simulink model "TestRoomVolume"  (R2025b)
settings: Solver=daessc  StartTime=0.0  StopTime=7200  FixedStep=3600  MaxStep=3  RelTol=1e-3  AbsTol=1e-3
PreLoadFcn:
  | WallModelParams
libraries: fl_lib x3, nesl_utility x2, buildingEnergy_lib x1
CloseFcn:
  | clear flow out roomHeight wall win
settings Model: Creator=vikrants  LastModifiedBy=skota
settings SolverCC: AutoScaleAbsTol=off  AlgebraicLoopSolver=TrustRegion  MaxZcPerStep=1.0
settings DebuggingCC: UnconnectedInputMsg=warning  UnconnectedOutputMsg=warning  UnconnectedLineMsg=warning  SymbolicDimsDataTypeCodeGenerationDiagnostic=none
settings ModelReferenceCC: EnableRefExpFcnMdlSchedulingChecks=on
settings SFSimCC: CustomCodeUndefinedFunction=UseInterfaceOnly
settings RTWCC: GPUComputeCapability=3.5  DLArmComputeVersion=19.05
settings SimscapeCC: SimscapeLogType=all  SimscapeLogSimulationStatistics=on  SimscapeLogDataHistory=10000.0

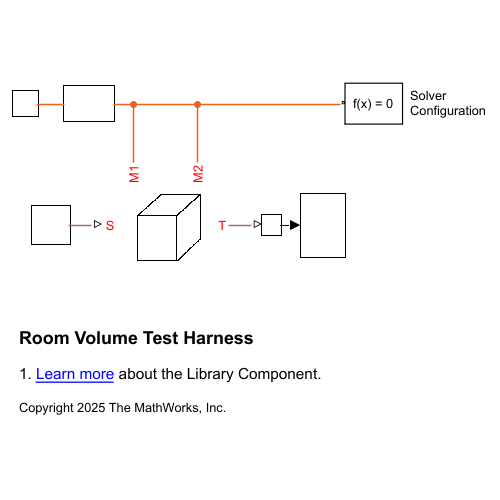
[thumbnail: Simulink's stored preview of the top-level diagram]
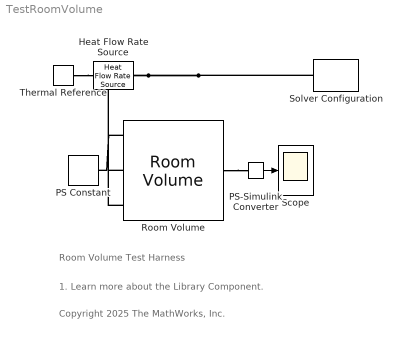
== system TestRoomVolume ==
  note: Room Volume Test Harness
  note: 1. Learn more about the Library Component.
  note: Copyright 2025 The MathWorks, Inc.
  Heat Flow Rate Source : fl_lib/Thermal/Thermal Sources/Heat Flow Rate Source  heat_flow=100 W
  PS Constant : fl_lib/Physical Signals/Sources/PS Constant  constant=100 J/s
  PS-Simulink Converter : nesl_utility/PS-Simulink Converter  PhysicalDomain=network_engine_domain  SubClassName=ps_output  LeftPortType=input  RightPortType=output  PseudoPeriodic=off  Frequencies=[]  VectorFormat=inherit  Unit=inherit  AffineConversion=off
  Room Volume : buildingEnergy_lib/Room Volume  N1=1  N2=1  iniT=300 K  length=5 m  width=3 m  height=2.5 m
  Scope : Scope
      settings: ActiveDisplayYMinimum=294.54266386219956  ActiveDisplayYMaximum=349.11602524020395
  Solver Configuration : nesl_utility/Solver Configuration  PhysicalDomain=network_engine_domain  SubClassName=solver  LeftPortType=input  RightPortType=generic  Tones=[]  Harmonics=[]  SimulateNoise=off  Profile=off  UseLocalSampling=off  EnableSwitchedLinearOptims=on  FrequencyDomain=off  UseCCode=off  RelTol=0.001  AbsTol=1e-06  MinStep=1e-09  ToWorkspace=off  RevertToSquareIcSolve=off  NumHomotopyIterations=100  PhasorMode=off  PhasorModeNumHarmonics=1  ConsistencySolver=NEWTON_XTOL_AFTER_FTOL  CanonicalOrdering=UNORDERED  OptimizeIntermediates=UNOPTIMIZED  IndexReductionMethod=DerivativeReplacement  DoDC=off  ResidualTolerance=1e-09  ConsistencyTolSource=GLOBAL  ConsistencyAbsTol=0.001  ConsistencyRelTol=0.001  ConsistencyTolFactor=0.001  UseLocalSolver=off  LocalSolverChoice=NE_BACKWARD_EULER_ADVANCER  ResolveIndetEquations=on  FunctionEvalNumThread=1  LocalSolverSampleTime=0.001  DoFixedCost=off  MaxNonlinIter=3  MaxModeIter=2  ComputeImpulses=off  ImpulseIterations=2  LinearAlgebra=auto  LinearAlgebraNumThread=0  EquationFormulation=NE_TIME_EF  DelaysMemoryBudget=1024  AutomaticFiltering=on  FilteringTimeConstant=0.001  PartitionStorageMethod=AS_NEEDED  PartitionMemoryBudget=1024  PartitionMethod=ROBUST  MultibodyUseLocalSolver=off  MultibodyLocalSolverChoice=ODE1  MultibodyLocalSolverSampleTime=0.001
  Thermal Reference : fl_lib/Thermal/Thermal Elements/Thermal Reference
  wires:
  PS-Simulink Converter/1 -> Scope/1
  connections:
  Thermal Reference/LConn1 -- Heat Flow Rate Source/RConn1
  Solver Configuration/RConn1 -- Room Volume/LConn3 -- Room Volume/LConn2 -- Heat Flow Rate Source/LConn1
  Room Volume/LConn1 -- PS Constant/RConn1
  Room Volume/RConn1 -- PS-Simulink Converter/LConn1
